simulink model "SAS_Simulation_A320"  (R2025b)
settings: Solver=ode15s  StartTime=0.0  StopTime=100  MaxStep=1e-4  RelTol=1e-5
values from neighbouring files (symbols this model uses):
  F_p = zeros(length(theta_deg), length(Vel))    [Load.m]    (also in SAS_Load_A320.m; saa_load_a320_v1.m)
  theta_deg = linspace(-25, 25, 100)    [AI_gen_code.m]    (also in AI_gen_code_2.m; Displacement_vsDeflection_angle_the_real_one.m = linspace(theta_min_deg,theta_max_deg,100); Geometry.m = linspace(theta_min_deg,theta_max_deg,101); SAS_Geometry_A320.m = linspace(theta_min_deg,theta_max_deg,101))
  Vel = linspace(vel_min, vel_max, 101)    [Load.m]    (also in SAS_Load_A320.m; saa_load_a320_v1.m)
  x = P-Po    [Displacement_vsDeflection_angle_the_real_one.m]    (also in Geometry.m = P - Po; SAS_Geometry_A320.m = P - Po; initial_geometry.m = 1:length(dalpha); sas_geometry_a320_v1.m = P - Po)
libraries: simulink x2, slpidlib x1
settings Model: Creator=mykha  LastModifiedBy=mykha
settings DebuggingCC: AlgebraicLoopMsg=none

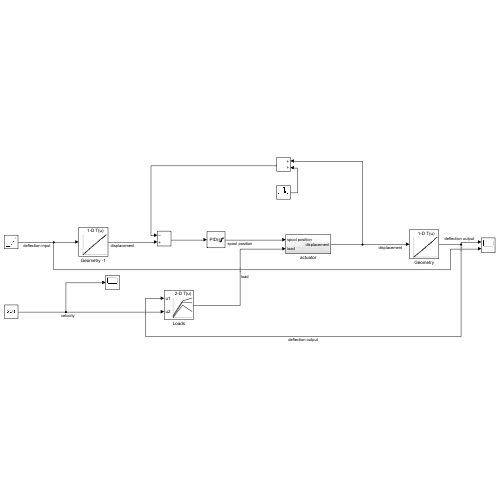
[thumbnail: Simulink's stored preview of the top-level diagram]
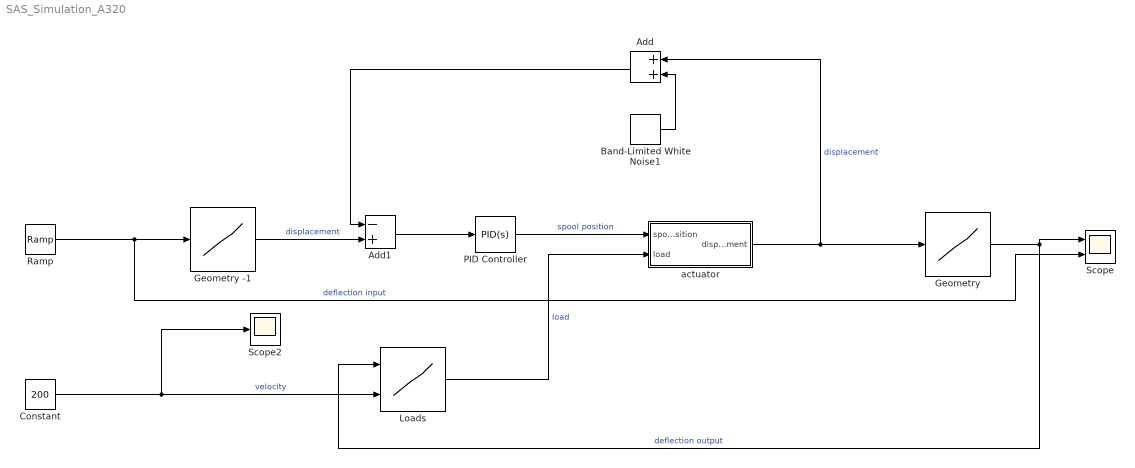
== system SAS_Simulation_A320 ==
  Add : Sum
  Add1 : Sum  Inputs=-+
  Band-Limited White Noise1 : simulink/Sources/Band-Limited White Noise  Cov=[1e-6]  Ts=0.1  seed=[23341]
  Constant : Constant  Value=200
  Geometry : Lookup_n-D  NumberOfTableDimensions=1  BreakpointsForDimension1=x  Table=theta_deg  InternalRulePriority=Speed  RndMeth=Simplest
  Geometry -1 : Lookup_n-D  NumberOfTableDimensions=1  BreakpointsForDimension1=theta_deg  Table=x  InternalRulePriority=Speed  RndMeth=Simplest
  Loads : Lookup_n-D  BreakpointsForDimension1=theta_deg  BreakpointsForDimension2=Vel  Table=F_p  InternalRulePriority=Speed  RndMeth=Simplest
      settings: InputPortMap=u0,u1
  PID Controller : slpidlib/PID Controller  Controller=PID  Form=Parallel  TimeDomain=Continuous-time  UseExternalTs=off  SampleTime=-1  IntegratorMethod=Forward Euler  FilterMethod=Forward Euler  ControllerParametersSource=internal  P=1.65170829982776  I=1.08207434366582  UseKiTs=off  D=0.237039060253964  UseExternalDerivativeSource=off  N=2.34008773826101  UseFilter=on  TunerSelectOption=Transfer Function Based (PID Tuner App)  InitialConditionSource=internal  InitialConditionForIntegrator=0  InitialConditionForFilter=0  DifferentiatorICPrevScaledInput=0  ExternalReset=none  TrackingMode=off  Kt=1  LimitOutput=on  SatLimitsSource=internal  UpperSaturationLimit=1  LowerSaturationLimit=-1  LinearizeAsGain=on  AntiWindupMode=none  Kb=1  LimitIntegrator=off  UpperIntegratorSaturationLimit=inf  LowerIntegratorSaturationLimit=-inf  POutMin=[]  POutMax=[]  IOutMin=[]  IOutMax=[]  DOutMin=[]  DOutMax=[]  NOutMin=[]  NOutMax=[]  SumOutMin=[]  SumOutMax=[]  SaturationOutMin=[]  SaturationOutMax=[]  PParamMin=[]  PParamMax=[]  IParamMin=[]  IParamMax=[]  DParamMin=[]  DParamMax=[]  NParamMin=[]  NParamMax=[]  KbParamMin=[]  KbParamMax=[]  KtParamMin=[]  KtParamMax=[]  KbOutMin=[]  KbOutMax=[]  KtOutMin=[]  KtOutMax=[]  IntegratorOutMin=[]  IntegratorOutMax=[]  FilterOutMin=[]  FilterOutMax=[]  SumI1OutMin=[]  SumI1OutMax=[]  SumI2OutMin=[]  SumI2OutMax=[]  SumI3OutMin=[]  SumI3OutMax=[]  SumI4OutMin=[]  SumI4OutMax=[]  SumDOutMin=[]  SumDOutMax=[]  DifferentiatorOutMin=[]  DifferentiatorOutMax=[]  FilterDiffOutCoefMin=[]  FilterDiffOutCoefMax=[]  ReciprocalOutMin=[]  ReciprocalOutMax=[]  SumDenOutMin=[]  SumDenOutMax=[]  SumNumOutMin=[]  SumNumOutMax=[]  DivideOutMin=[]  DivideOutMax=[]  UdiffTsProdOutMin=[]  UdiffTsProdOutMax=[]  NTsProdOutMin=[]  NTsProdOutMax=[]  UintegralTsProdOutMin=[]  UintegralTsProdOutMax=[]  UngainTsProdOutMin=[]  UngainTsProdOutMax=[]  ClampingZeroOutDataTypeStr=Inherit: Inherit via back propagation  ClampingZeroOutMin=[]  ClampingZeroOutMax=[]  FilterDenConstantOutDataTypeStr=Inherit: Inherit via back propagation  FilterDenConstantOutMin=[]  FilterDenConstantOutMax=[]  PCopyOutDataTypeStr=Inherit: Inherit via back propagation  PCopyOutMin=[]  PCopyOutMax=[]  NCopyOutDataTypeStr=Inherit: Inherit via back propagation  NCopyOutMin=[]  NCopyOutMax=[]  IntegratorContinuousStateAttributes=''  IntegratorStateMustResolveToSignalObject=off  IntegratorRTWStateStorageClass=Auto  FilterContinuousStateAttributes=''  FilterStateMustResolveToSignalObject=off  FilterRTWStateStorageClass=Auto  ParallelPVariant=InternalParameters  IdealPVariant=Disabled  IVariant=InternalParameters  DVariant=InternalParameters  IntegratorVariant=Continuous  SatVariant=Enabled  AWVariant=Passthrough  PCopyVariant=Disabled  TRVariant=Disabled  FdbkBlocksVariant=Forward  IdealPFdbkVariant=Disabled  SatFdbkVariant=Disabled  DerivativeFilterVariant=ContFilter  NVariant=InternalParameters  NCopyVariant=Disabled  FilterICVariant=InternalICsFilter  IntegratorICVariant=InternalICs  ExternalResetVariant=Disabled  TRSumVariant=Passthrough  SumFdbkVariant=Disabled  SumVariant=Sum_PID  TsampFilterVariant=InternalTs  TsampNgainVariant=Passthrough  TsampIntegralVariant=Disabled_SignalSpec  ExternalSaturationOutDataTypeStr=Inherit: Same as second input  DerivativeSourceVariant=ErrorSignal  PreIntVariant=InternalPreInt
  Ramp : simulink/Sources/Ramp  slope=0.3  start=0  InitialOutput=-15
  Scope : Scope  NumInputPorts=2
      settings: ActiveDisplayYMinimum=-34.469365151660284  ActiveDisplayYMaximum=43.552468977729724
  Scope2 : Scope
      settings: ActiveDisplayYMinimum=102.28012454025719  ActiveDisplayYMaximum=229.47887913768528  DataLoggingVariableName=ScopeData3
  actuator : Subsystem
  wires:
  Ramp/1 -> Scope/2, Geometry -1/1  "deflection input"
  Geometry -1/1 -> Add1/2  "displacement"
  Geometry/1 -> Scope/1, Loads/1  "deflection output"
  PID Controller/1 -> actuator/1(spool position)  "spool position"
  Loads/1 -> actuator/2(load)  "load"
  actuator/1(displacement) -> Geometry/1, Add/1  "displacement"
  Add1/1 -> PID Controller/1
  Constant/1 -> Scope2/1, Loads/2  "velocity"
  Add/1 -> Add1/1
  Band-Limited White Noise1/1 -> Add/2

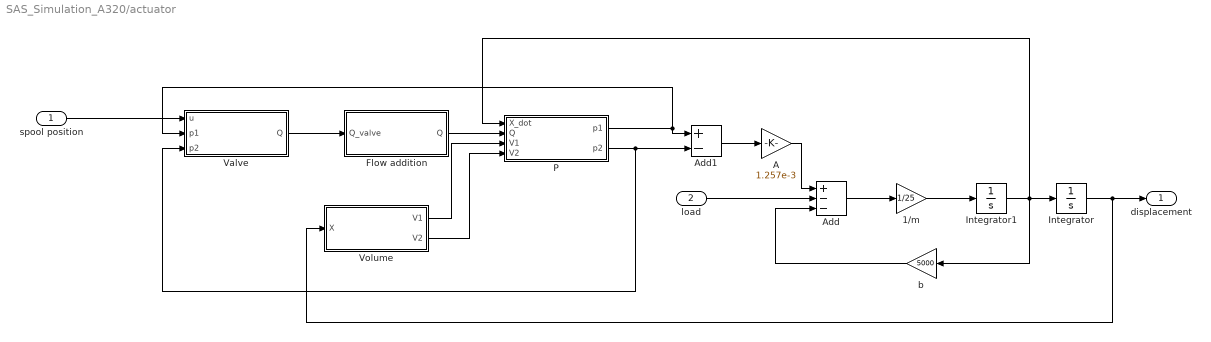
== system SAS_Simulation_A320/actuator ==
  spool position : Inport
  load : Inport  Port=2
  1/m : Gain  Gain=1/25
  A : Gain  Gain=1.257e-3
  Add : Sum  Inputs=+--
  Add1 : Sum  Inputs=+-
  Flow addition : Subsystem
  Integrator : Integrator
  Integrator1 : Integrator
  P : Subsystem
  Valve : Subsystem
  Volume : Subsystem
  b : Gain  Gain=5000
  displacement : Outport
  wires:
  spool position/1 -> Valve/1(u)
  P/2(p2) -> Add1/2, Valve/3(p2)
  P/1(p1) -> Add1/1, Valve/2(p1)
  Integrator1/1 -> Integrator/1, b/1, P/1(X_dot)
  Integrator/1 -> displacement/1, Volume/1(X)
  Volume/1(V1) -> P/3(V1)
  Volume/2(V2) -> P/4(V2)
  1/m/1 -> Integrator1/1
  Add/1 -> 1/m/1
  load/1 -> Add/2
  Add1/1 -> A/1
  A/1 -> Add/1
  b/1 -> Add/3
  Valve/1(Q) -> Flow addition/1(Q_valve)
  Flow addition/1(Q) -> P/2(Q)

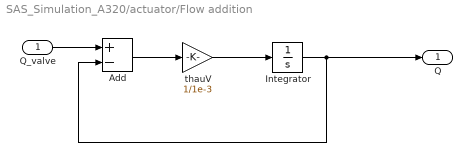
== system SAS_Simulation_A320/actuator/Flow addition ==
  Q_valve : Inport
  Add : Sum  Inputs=+-
  Integrator : Integrator
  thauV : Gain  Gain=1/1e-3
  Q : Outport
  wires:
  Q_valve/1 -> Add/1
  Add/1 -> thauV/1
  thauV/1 -> Integrator/1
  Integrator/1 -> Q/1, Add/2

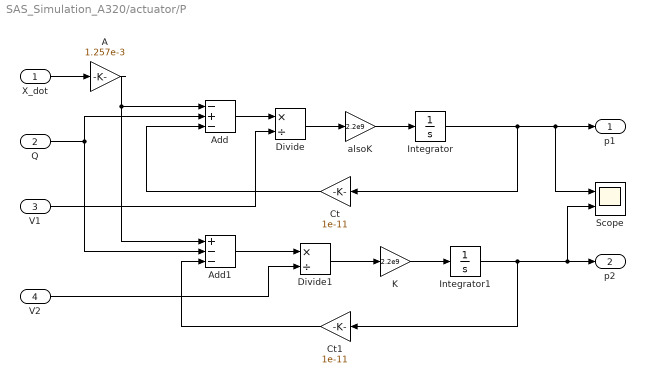
== system SAS_Simulation_A320/actuator/P ==
  X_dot : Inport
  Q : Inport  Port=2
  V1 : Inport  Port=3
  V2 : Inport  Port=4
  A : Gain  Gain=1.257e-3
  Add : Sum  Inputs=-+-
  Add1 : Sum  Inputs=+--
  Ct : Gain  Gain=1e-11
  Ct1 : Gain  Gain=1e-11
  Divide : Product  Inputs=*/
  Divide1 : Product  Inputs=*/
  Integrator : Integrator
  Integrator1 : Integrator
  K : Gain  Gain=2.2e9
  Scope : Scope  NumInputPorts=2
      settings: ActiveDisplayYMinimum=-6.1931291268066317E+6  ActiveDisplayYMaximum=6.192675425209973E+6
  alsoK : Gain  Gain=2.2e9
  p1 : Outport
  p2 : Outport  Port=2
  wires:
  alsoK/1 -> Integrator/1
  A/1 -> Add1/1, Add/1
  Q/1 -> Add/2, Add1/2
  Add/1 -> Divide/1
  Divide/1 -> alsoK/1
  V1/1 -> Divide/2
  Add1/1 -> Divide1/1
  V2/1 -> Divide1/2
  Divide1/1 -> K/1
  K/1 -> Integrator1/1
  X_dot/1 -> A/1
  Integrator1/1 -> Scope/2, p2/1, Ct1/1
  Integrator/1 -> Ct/1, Scope/1, p1/1
  Ct/1 -> Add/3
  Ct1/1 -> Add1/3

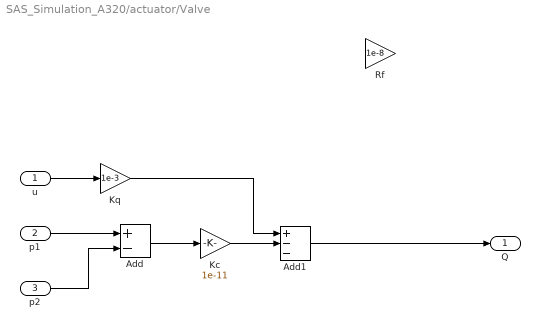
== system SAS_Simulation_A320/actuator/Valve ==
  u : Inport
  p1 : Inport  Port=2
  p2 : Inport  Port=3
  Add : Sum  Inputs=+-
  Add1 : Sum  Inputs=+--
  Kc : Gain  Gain=1e-11
  Kq : Gain  Gain=1e-3
  Rf : Gain  Gain=1e-8
  Q : Outport
  wires:
  p1/1 -> Add/1
  p2/1 -> Add/2
  u/1 -> Kq/1
  Kq/1 -> Add1/1
  Add/1 -> Kc/1
  Add1/1 -> Q/1
  Kc/1 -> Add1/2

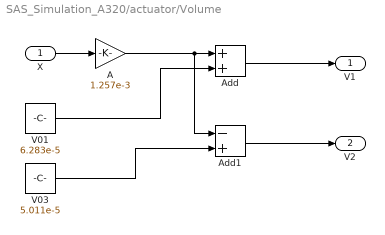
== system SAS_Simulation_A320/actuator/Volume ==
  X : Inport
  A : Gain  Gain=1.257e-3
  Add : Sum
  Add1 : Sum  Inputs=-+
  V01 : Constant  Value=6.283e-5
  V03 : Constant  Value=5.011e-5
  V1 : Outport
  V2 : Outport  Port=2
  wires:
  X/1 -> A/1
  A/1 -> Add/1, Add1/1
  Add/1 -> V1/1
  Add1/1 -> V2/1
  V01/1 -> Add/2
  V03/1 -> Add1/2
